simulink model "six_plus_six_AcmsteeringV10_main"  (R2014a)
settings: Solver=FixedStepDiscrete  StartTime=0.0  StopTime=10.0  FixedStep=0.0005  RelTol=1e-3
InitFcn:
  | Veh_Par_wxt
values from neighbouring files (symbols this model uses):
  acc_spdctl = [0 100]    [Veh_Par_wxt.m]
  ag_thr = ecucoder_cal(ag_thr)    [Veh_Par_wxt.m]
  B = 1.8    [Veh_Par_wxt.m]
  bra_em = 100    [Veh_Par_wxt.m]
  bra_pre_gz2 = 100/3    (= 33.3333333333)    [Veh_Par_wxt.m]
  bra_pre_gz34 = 10/3    (= 3.33333333333)    [Veh_Par_wxt.m]
  bra_pre_yd = 10/2    (= 5)    [Veh_Par_wxt.m]
  brakepre_dem_data = [0 1 2 3 4 5 6 7 8 9 10]    [Veh_Par_wxt.m]
  brakeTrq_dem_data = [0 125 251 376 502 627 753 878 1004 1129 1255]    [Veh_Par_wxt.m]
  bratrq_max = 4*1255    (= 5020)    [Veh_Par_wxt.m]
  eff_tran = 0.9    [Veh_Par_wxt.m]
  ESP_switch = ecucoder_cal(ESP_switch)    [Veh_Par_wxt.m]
  G = Mass*g    (= 15696)    [Veh_Par_wxt.m]
  kd1 = ecucoder_cal(kd1)    [Veh_Par_wxt.m]
  kd2 = 0    [Veh_Par_wxt.m]
  ki1 = ecucoder_cal(ki1)    [Veh_Par_wxt.m]
  ki2 = 1    [Veh_Par_wxt.m]
  kp1 = ecucoder_cal(kp1)    [Veh_Par_wxt.m]
  kp2 = 300    [Veh_Par_wxt.m]
  L = L1+L2    (= 2.9)    [Veh_Par_wxt.m]
  premax = 100    [Veh_Par_wxt.m]
  Radius = 0.4572/2    (= 0.2286)    [Veh_Par_wxt.m]
  RC_switch = ecucoder_cal(RC_switch)    [Veh_Par_wxt.m]
  s_opt_yi = 0.15    [Veh_Par_wxt.m]
  s_opt_zhuan = 0.8    [Veh_Par_wxt.m]
  s_opt_zhuan_add = 0.05    [Veh_Par_wxt.m]
  s_opt_zhuan_table = [0.8 0.8 0.3 0.3]    [Veh_Par_wxt.m]
  spd_map_mot = [0 499.85 999.79 1500 2000 2500 3000 3500 4000 4500 4999.8 5999.8]    [Veh_Par_wxt.m]
  spd_spdctl = [0 500]    [Veh_Par_wxt.m]
  speed_thr_park = 5/3.6/Radius*tras_ratio*30/pi    (= 464.143899364)    [Veh_Par_wxt.m]
  TCS_switch = ecucoder_cal(TCS_switch)    [Veh_Par_wxt.m]
  tras_ratio = 8    [Veh_Par_wxt.m]
  trq_map_mot = [70.5 70.012 71.154 65.797 53.917 45.159 38.073 32.685 27.48 17.133 14.949 10.07]    [Veh_Par_wxt.m]
  trqmax_yd = 70.5    [Veh_Par_wxt.m]
  trqmax_zx = 70.5    [Veh_Par_wxt.m]
  trqmaxneg = -70.5    [Veh_Par_wxt.m]
  v_gain = 0.9    [Veh_Par_wxt.m]
  v_table = [0 5 20 100]    [Veh_Par_wxt.m]
  v_thr_park = 5    [Veh_Par_wxt.m]
  zhidong_bianmazhi = [-140000 750000]    [Veh_Par_wxt.m]
  zhidong_down = -140000    [Veh_Par_wxt.m]
  zhidong_up = 750000    [Veh_Par_wxt.m]
  zhidong_youmen = [0 100]    [Veh_Par_wxt.m]
  zhuanxiang_bianmazhi = [-400000 0 400000]    [Veh_Par_wxt.m]
  zhuanxiang_down = -400000    [Veh_Par_wxt.m]
  zhuanxiang_up = 400000    [Veh_Par_wxt.m]
  zhuanxiang_youmen = [-100 0 100]    [Veh_Par_wxt.m]
undefined symbols (not defined in the file or in its folder): ecucoder_acal, guzhang_lf, guzhang_lm, guzhang_lr, guzhang_rf, guzhang_rm, guzhang_rr, myFIS
libraries: simulink x979, ec5744lib x59, fuzblock x2
(part 26 of 27)

== system six_plus_six_AcmsteeringV10_main/MainControl/mode_control/backward/backward/Drive/驱动防滑控制TCS/直行TCS/直行/Subsystem/Subsystem5 ==
  s_opt_zhuan : Inport
  s_act_rm : Inport  Port=2
  trq_dem_rm : Inport  Port=3
  Action Port : ActionPort  InitializeStates=reset  ActionType=then
  Add11 : Sum  Inputs=+++
  Add8 : Sum  AccumDataTypeStr=single
  Add9 : Sum  Inputs=+-+
  Data Type Conversion2 : DataTypeConversion
  Gain14 : Gain  Gain=1/tras_ratio  OutDataTypeStr=Inherit: Inherit via back propagation
  Gain16 : Gain  Gain=kp2  OutDataTypeStr=single
  Gain17 : Gain  Gain=ki2  OutDataTypeStr=single
  Gain18 : Gain  Gain=2
  Gain19 : Gain  Gain=kd2  OutDataTypeStr=single
  Memory{1..2,6,15} (4 alike) : Memory  InheritSampleTime=on
  Saturation : Saturate  UpperLimit=inf  LowerLimit=0
  Subtract2 : Sum  Inputs=+-
  Subtract7 : Sum
  Sum3 : Sum  Inputs=|+-
  trq_pid_rm : Outport
  wires:
  Saturation/1 -> Data Type Conversion2/1
  Subtract7/1 -> Gain14/1, Memory15/1
  Data Type Conversion2/1 -> trq_pid_rm/1
  Add11/1 -> Subtract7/1
  Memory15/1 -> Subtract7/2
  Gain18/1 -> Add9/2
  Memory2/1 -> Gain18/1, Memory6/1
  Sum3/1 -> Memory1/1, Gain17/1, Add9/1, Memory2/1, Subtract2/1
  s_opt_zhuan/1 -> Sum3/1
  Add8/1 -> Saturation/1
  Gain16/1 -> Add11/1
  Memory6/1 -> Add9/3
  Gain19/1 -> Add11/3
  Gain14/1 -> Add8/1
  Gain17/1 -> Add11/2
  Add9/1 -> Gain19/1
  Subtract2/1 -> Gain16/1
  s_act_rm/1 -> Sum3/2
  Memory1/1 -> Subtract2/2
  trq_dem_rm/1 -> Add8/2

== system six_plus_six_AcmsteeringV10_main/MainControl/mode_control/forward/forward/Drive/驱动防滑控制TCS/直行TCS/直行/Subsystem/Subsystem ==
  s_opt_zhuan : Inport
  s_act_lf : Inport  Port=2
  trq_dem_lf : Inport  Port=3
  Action Port : ActionPort  InitializeStates=reset  ActionType=then
  Add10 : Sum  Inputs=+-+
  Add2 : Sum  Inputs=+++
  Add3 : Sum  AccumDataTypeStr=single
  Data Type Conversion : DataTypeConversion
  Gain : Gain  Gain=1/tras_ratio  OutDataTypeStr=Inherit: Inherit via back propagation
  Gain1 : Gain  Gain=kp2  OutDataTypeStr=single
  Gain2 : Gain  Gain=ki2  OutDataTypeStr=single
  Gain20 : Gain  Gain=2
  Gain3 : Gain  Gain=kd2  OutDataTypeStr=single
  Memory{3..5,13} (4 alike) : Memory  InheritSampleTime=on
  Saturation : Saturate  UpperLimit=inf  LowerLimit=0
  Subtract1 : Sum  Inputs=+-
  Subtract5 : Sum
  Sum : Sum  Inputs=|+-
  trq_pid_lf : Outport
  wires:
  trq_dem_lf/1 -> Add3/2
  s_act_lf/1 -> Sum/2
  Add3/1 -> Saturation/1
  Sum/1 -> Subtract1/1, Memory4/1, Add10/1, Gain2/1, Memory3/1
  Gain/1 -> Add3/1  "trq_pid_lf_adjust"
  s_opt_zhuan/1 -> Sum/1
  Gain1/1 -> Add2/1
  Gain2/1 -> Add2/2
  Memory3/1 -> Subtract1/2
  Add10/1 -> Gain3/1
  Gain20/1 -> Add10/2
  Memory5/1 -> Add10/3
  Gain3/1 -> Add2/3
  Subtract1/1 -> Gain1/1
  Memory4/1 -> Memory5/1, Gain20/1
  Add2/1 -> Subtract5/1
  Subtract5/1 -> Memory13/1, Gain/1
  Memory13/1 -> Subtract5/2
  Data Type Conversion/1 -> trq_pid_lf/1
  Saturation/1 -> Data Type Conversion/1

== system six_plus_six_AcmsteeringV10_main/MainControl/mode_control/forward/forward/Drive/驱动防滑控制TCS/直行TCS/直行/Subsystem/Subsystem1 ==
  s_opt_zhuan : Inport
  s_act_lr : Inport  Port=2
  trq_dem_lr : Inport  Port=3
  Action Port : ActionPort  InitializeStates=reset  ActionType=then
  Add10 : Sum  Inputs=+-+
  Add2 : Sum  Inputs=+++
  Add3 : Sum  AccumDataTypeStr=single
  Data Type Conversion : DataTypeConversion
  Gain : Gain  Gain=1/tras_ratio  OutDataTypeStr=Inherit: Inherit via back propagation
  Gain1 : Gain  Gain=kp2  OutDataTypeStr=single
  Gain2 : Gain  Gain=ki2  OutDataTypeStr=single
  Gain20 : Gain  Gain=2
  Gain3 : Gain  Gain=kd2  OutDataTypeStr=single
  Memory{3..5,13} (4 alike) : Memory  InheritSampleTime=on
  Saturation : Saturate  UpperLimit=inf  LowerLimit=0
  Subtract1 : Sum  Inputs=+-
  Subtract5 : Sum
  Sum : Sum  Inputs=|+-
  trq_pid_lr : Outport
  wires:
  trq_dem_lr/1 -> Add3/2
  s_act_lr/1 -> Sum/2
  Add3/1 -> Saturation/1
  Sum/1 -> Subtract1/1, Memory4/1, Add10/1, Gain2/1, Memory3/1
  Gain/1 -> Add3/1  "trq_pid_lr_adjust"
  s_opt_zhuan/1 -> Sum/1
  Gain1/1 -> Add2/1
  Gain2/1 -> Add2/2
  Memory3/1 -> Subtract1/2
  Add10/1 -> Gain3/1
  Gain20/1 -> Add10/2
  Memory5/1 -> Add10/3
  Gain3/1 -> Add2/3
  Subtract1/1 -> Gain1/1
  Memory4/1 -> Memory5/1, Gain20/1
  Add2/1 -> Subtract5/1
  Subtract5/1 -> Gain/1, Memory13/1
  Memory13/1 -> Subtract5/2
  Data Type Conversion/1 -> trq_pid_lr/1
  Saturation/1 -> Data Type Conversion/1

== system six_plus_six_AcmsteeringV10_main/MainControl/mode_control/forward/forward/Drive/驱动防滑控制TCS/直行TCS/直行/Subsystem/Subsystem2 ==
  s_opt_zhuan : Inport
  s_act_rf : Inport  Port=2
  trq_dem_rf : Inport  Port=3
  Action Port : ActionPort  InitializeStates=reset  ActionType=then
  Add11 : Sum  Inputs=+++
  Add8 : Sum  AccumDataTypeStr=single
  Add9 : Sum  Inputs=+-+
  Data Type Conversion2 : DataTypeConversion
  Gain14 : Gain  Gain=1/tras_ratio  OutDataTypeStr=Inherit: Inherit via back propagation
  Gain16 : Gain  Gain=kp2  OutDataTypeStr=single
  Gain17 : Gain  Gain=ki2  OutDataTypeStr=single
  Gain18 : Gain  Gain=2
  Gain19 : Gain  Gain=kd2  OutDataTypeStr=single
  Memory{1..2,6,15} (4 alike) : Memory  InheritSampleTime=on
  Saturation : Saturate  UpperLimit=inf  LowerLimit=0
  Subtract2 : Sum  Inputs=+-
  Subtract7 : Sum
  Sum3 : Sum  Inputs=|+-
  trq_pid_rf : Outport
  wires:
  trq_dem_rf/1 -> Add8/2
  Memory1/1 -> Subtract2/2
  s_act_rf/1 -> Sum3/2
  Subtract2/1 -> Gain16/1
  Add9/1 -> Gain19/1
  Gain17/1 -> Add11/2
  Gain14/1 -> Add8/1  "trq_pid_rf_adjust"
  Gain19/1 -> Add11/3
  Memory6/1 -> Add9/3
  Gain16/1 -> Add11/1
  Add8/1 -> Saturation/1
  s_opt_zhuan/1 -> Sum3/1
  Sum3/1 -> Subtract2/1, Memory2/1, Add9/1, Gain17/1, Memory1/1
  Memory2/1 -> Memory6/1, Gain18/1
  Gain18/1 -> Add9/2
  Memory15/1 -> Subtract7/2
  Add11/1 -> Subtract7/1
  Data Type Conversion2/1 -> trq_pid_rf/1
  Subtract7/1 -> Memory15/1, Gain14/1
  Saturation/1 -> Data Type Conversion2/1

== system six_plus_six_AcmsteeringV10_main/MainControl/mode_control/forward/forward/Drive/驱动防滑控制TCS/直行TCS/直行/Subsystem/Subsystem3 ==
  s_opt_zhuan : Inport
  s_act_rr : Inport  Port=2
  trq_dem_rr : Inport  Port=3
  Action Port : ActionPort  InitializeStates=reset  ActionType=then
  Add12 : Sum  Inputs=+-+
  Add13 : Sum  Inputs=+++
  Add6 : Sum  AccumDataTypeStr=single
  Data Type Conversion3 : DataTypeConversion
  Gain15 : Gain  Gain=1/tras_ratio  OutDataTypeStr=Inherit: Inherit via back propagation
  Gain21 : Gain  Gain=kp2  OutDataTypeStr=single
  Gain22 : Gain  Gain=ki2  OutDataTypeStr=single
  Gain23 : Gain  Gain=2
  Gain24 : Gain  Gain=kd2  OutDataTypeStr=single
  Memory{7..9,16} (4 alike) : Memory  InheritSampleTime=on
  Saturation : Saturate  UpperLimit=inf  LowerLimit=0
  Subtract3 : Sum  Inputs=+-
  Subtract8 : Sum
  Sum2 : Sum  Inputs=|+-
  trq_pid_rr : Outport
  wires:
  trq_dem_rr/1 -> Add6/2
  s_act_rr/1 -> Sum2/2
  Add6/1 -> Saturation/1
  s_opt_zhuan/1 -> Sum2/1
  Sum2/1 -> Memory8/1, Add12/1, Gain22/1, Memory7/1, Subtract3/1
  Gain15/1 -> Add6/1  "trq_pid_rr_adjust"
  Gain21/1 -> Add13/1
  Add13/1 -> Subtract8/1
  Memory8/1 -> Memory9/1, Gain23/1
  Gain23/1 -> Add12/2
  Memory7/1 -> Subtract3/2
  Memory9/1 -> Add12/3
  Data Type Conversion3/1 -> trq_pid_rr/1
  Gain22/1 -> Add13/2
  Add12/1 -> Gain24/1
  Gain24/1 -> Add13/3
  Subtract3/1 -> Gain21/1
  Memory16/1 -> Subtract8/2
  Subtract8/1 -> Gain15/1, Memory16/1
  Saturation/1 -> Data Type Conversion3/1

== system six_plus_six_AcmsteeringV10_main/MainControl/mode_control/forward/forward/Drive/驱动防滑控制TCS/直行TCS/直行/Subsystem/Subsystem4 ==
  s_opt_zhuan : Inport
  s_act_lm : Inport  Port=2
  trq_dem_lm : Inport  Port=3
  Action Port : ActionPort  InitializeStates=reset  ActionType=then
  Add10 : Sum  Inputs=+-+
  Add2 : Sum  Inputs=+++
  Add3 : Sum  AccumDataTypeStr=single
  Data Type Conversion : DataTypeConversion
  Gain : Gain  Gain=1/tras_ratio  OutDataTypeStr=Inherit: Inherit via back propagation
  Gain1 : Gain  Gain=kp2  OutDataTypeStr=single
  Gain2 : Gain  Gain=ki2  OutDataTypeStr=single
  Gain20 : Gain  Gain=2
  Gain3 : Gain  Gain=kd2  OutDataTypeStr=single
  Memory{3..5,13} (4 alike) : Memory  InheritSampleTime=on
  Saturation : Saturate  UpperLimit=inf  LowerLimit=0
  Subtract1 : Sum  Inputs=+-
  Subtract5 : Sum
  Sum : Sum  Inputs=|+-
  trq_pid_lm : Outport
  wires:
  Saturation/1 -> Data Type Conversion/1
  Data Type Conversion/1 -> trq_pid_lm/1
  Memory13/1 -> Subtract5/2
  Subtract5/1 -> Gain/1, Memory13/1
  Add2/1 -> Subtract5/1
  Memory4/1 -> Gain20/1, Memory5/1
  Subtract1/1 -> Gain1/1
  Gain3/1 -> Add2/3
  Memory5/1 -> Add10/3
  Gain20/1 -> Add10/2
  Add10/1 -> Gain3/1
  Memory3/1 -> Subtract1/2
  Gain2/1 -> Add2/2
  Gain1/1 -> Add2/1
  s_opt_zhuan/1 -> Sum/1
  Gain/1 -> Add3/1  "trq_pid_lm_adjust"
  Sum/1 -> Memory3/1, Gain2/1, Add10/1, Memory4/1, Subtract1/1
  Add3/1 -> Saturation/1
  s_act_lm/1 -> Sum/2
  trq_dem_lm/1 -> Add3/2

== system six_plus_six_AcmsteeringV10_main/MainControl/mode_control/forward/forward/Drive/驱动防滑控制TCS/直行TCS/直行/Subsystem/Subsystem5 ==
  s_opt_zhuan : Inport
  s_act_rm : Inport  Port=2
  trq_dem_rm : Inport  Port=3
  Action Port : ActionPort  InitializeStates=reset  ActionType=then
  Add11 : Sum  Inputs=+++
  Add8 : Sum  AccumDataTypeStr=single
  Add9 : Sum  Inputs=+-+
  Data Type Conversion2 : DataTypeConversion
  Gain14 : Gain  Gain=1/tras_ratio  OutDataTypeStr=Inherit: Inherit via back propagation
  Gain16 : Gain  Gain=kp2  OutDataTypeStr=single
  Gain17 : Gain  Gain=ki2  OutDataTypeStr=single
  Gain18 : Gain  Gain=2
  Gain19 : Gain  Gain=kd2  OutDataTypeStr=single
  Memory{1..2,6,15} (4 alike) : Memory  InheritSampleTime=on
  Saturation : Saturate  UpperLimit=inf  LowerLimit=0
  Subtract2 : Sum  Inputs=+-
  Subtract7 : Sum
  Sum3 : Sum  Inputs=|+-
  trq_pid_rm : Outport
  wires:
  Saturation/1 -> Data Type Conversion2/1
  Subtract7/1 -> Gain14/1, Memory15/1
  Data Type Conversion2/1 -> trq_pid_rm/1
  Add11/1 -> Subtract7/1
  Memory15/1 -> Subtract7/2
  Gain18/1 -> Add9/2
  Memory2/1 -> Gain18/1, Memory6/1
  Sum3/1 -> Memory1/1, Gain17/1, Add9/1, Memory2/1, Subtract2/1
  s_opt_zhuan/1 -> Sum3/1
  Add8/1 -> Saturation/1
  Gain16/1 -> Add11/1
  Memory6/1 -> Add9/3
  Gain19/1 -> Add11/3
  Gain14/1 -> Add8/1  "trq_pid_rm_adjust"
  Gain17/1 -> Add11/2
  Add9/1 -> Gain19/1
  Subtract2/1 -> Gain16/1
  s_act_rm/1 -> Sum3/2
  Memory1/1 -> Subtract2/2
  trq_dem_rm/1 -> Add8/2

== matlab function six_plus_six_AcmsteeringV10_main/MainControl/mode_control/Park/park/HeartBeat ==
  data: life_pre input; life output
function life = fcn(life_pre)
%#codegen
life=single(life_pre+1);
if life>255
    life=single(0);
end
end

== matlab function six_plus_six_AcmsteeringV10_main/MainControl/mode_control/forward/forward/Drive/目标转向力矩确定模块/MATLAB Function2 ==
  data: umax input; delta_Tsteer_max output; G input; L input; B input; Radius input; Rturn_min_xy input
function delta_Tsteer_max = fcn(umax,G,L,B,Radius,Rturn_min_xy)
%#codegen

    delta_Fsteer_max=single(umax/(0.925+0.15*(Rturn_min_xy/B))*G*L/(2*B));
    delta_Tsteer_max=single(delta_Fsteer_max*Radius);
    
end

== matlab function six_plus_six_AcmsteeringV10_main/MainControl/mode_control/Park/park/HeartBeat1 ==
  data: life_pre input; life output
function life = fcn(life_pre)
%#codegen
life=single(life_pre+1);
if life>255
    life=single(0);
end
end

== matlab function six_plus_six_AcmsteeringV10_main/MainControl/mode_control/forward/forward/Drive/目标转向力矩确定模块/MATLAB Function ==
  data: steer_dem input; Rturn_min output; G input; L input; umax input; B input; Tpeak_L input; Tpeak_R input; eff_tran input; Radius input; f input
function Rturn_min = fcn(steer_dem,G,L,umax,B,Tpeak_L,Tpeak_R,eff_tran,Radius,f)
%#codegen
if steer_dem>0
    Rturn_min=single((G*L*umax/(4*B*(Tpeak_R*eff_tran/Radius-f*G/2))-0.925)/0.15*B);
else
    Rturn_min=single((G*L*umax/(4*B*(Tpeak_L*eff_tran/Radius-f*G/2))-0.925)/0.15*B);
end
end

== matlab function six_plus_six_AcmsteeringV10_main/MainControl/mode_control/forward/forward/Drive/目标转向力矩确定模块/MATLAB Function1 ==
  data: v_act input; Rturn_min_ag output; ag_thr input
 function Rturn_min_ag = fcn(v_act,ag_thr)
%#codegen

    Rturn_min_ag=single((v_act/3.6)^2/ag_thr);
end

== matlab function six_plus_six_AcmsteeringV10_main/Data_input/181/Enabled
Subsystem/MATLAB Function3 ==
  data: speed input; speed_out output
function speed_out = motec_speed(speed)
    if speed>32768
        speed_out=speed-65535;
    else speed_out=speed;
    end
end

== matlab function six_plus_six_AcmsteeringV10_main/MainControl/mode_control/forward/forward/Drive/驱动防滑控制TCS/直行TCS/直行/HeartBeat2 ==
  data: life_pre input; life output
function life = fcn(life_pre)
%#codegen
life=single(life_pre+1);
if life>255
    life=single(0);
end
end

== matlab function six_plus_six_AcmsteeringV10_main/MainControl/mode_control/forward/forward/Drive/左右侧电机分配及功率限制/MATLAB Function ==
  data: trqlim_l input; trq_dem_l output; trq_dem_r output; trq_dem_l1 input; trqlim_r input; trq_dem_r1 input; delta_T_dem input
function [trq_dem_l,trq_dem_r] = fcn(trqlim_l,trq_dem_l1,trqlim_r,trq_dem_r1,delta_T_dem)
%#codegen
if trq_dem_l1==trqlim_l
    trq_dem_l=single(trq_dem_l1);
    trq_dem_r=single(trq_dem_l1+delta_T_dem);%这时候加的是负值
elseif trq_dem_r1==trqlim_r
    trq_dem_l=single(trq_dem_r1-delta_T_dem);
    trq_dem_r=single(trq_dem_r1);
    
else
    trq_dem_l=single(trq_dem_l1);
    trq_dem_r=single(trq_dem_r1);
end
% trq_dem_l=single(max(0,trq_dem_l));%限一下最小值，不要小于0
% trq_dem_r=single(max(0,trq_dem_r));
trq_dem_l=single(max(-trqlim_l,trq_dem_l));%小转向半径下，内侧履带是可能输出负转矩的，从地面吸收功率，给外侧，所以不能限到0，限到最大电机外特性负值
trq_dem_r=single(max(-trqlim_r,trq_dem_r));
end
